simulink model "TestModeleMachineElectrique"  (Simulink 10.0)
settings: Solver=VariableStepAuto  StartTime=0.0  StopTime=10.0  RelTol=1e-3
values from neighbouring files (symbols this model uses):
  ess_coulombic_eff = 0.99    [Batteries.m]
  ess_max_ah_cap = 28    [Batteries.m]
  ess_module_number = 20    [Batteries.m]
  ess_r = [0.01266 0.00685	0.00644	0.00599	0.00587	0.00575	0.00568	0.00581	0.00623	0.00667  0.00635]    [Batteries.m]
  ess_soc = [0:.1:1]    [Batteries.m]
  ess_tau = 0.1    [Batteries.m]
  ess_voc = [12.5 12.8 13.1 13.3 13.4 13.4 13.5 13.6 13.7 13.9 14.2]    [Batteries.m]
  mc_eff_map = 0.01*[ 20	20	20	20	20	20	20	20	20	20	20	20	20	20	20	20	20	20	20	20	20 ... (first row only)    [MachineElectrique.m]
  mc_inertia = 0.0226    [MachineElectrique.m]
  mc_map_spd = [0 500 1000 1500 2000 2500 3000 4000 5000 6000 7000]*(2*pi)/60    [MachineElectrique.m]
  mc_max_trq = [512 508.1 504.2 500.3 496.3	492.4 488.5 480.7 472.8 465 0]    *4.448/3.281/12    [MachineElectrique.m]
  mc_min_trq = -1*[512 508.1 504.2 500.3 496.3	492.4 488.5 480.7 472.8 465 0]    *4.448/3.281/12    [MachineElectrique.m]
  SocInit = 0.8    [Batteries.m]
settings Model: Creator=szhang6_  LastModifiedBy=szhang6_
settings DataIOCC: SaveFormat=Dataset
settings OptimizationCC: LifeSpan=auto
settings DebuggingCC: UnderspecifiedInitializationDetection=Simplified  MergeDetectMultiDrivingBlocksExec=error  SFUnexpectedBacktrackingDiag=error  SFNoUnconditionalDefaultTransitionDiag=error  SFExecutionAtInitializationDiag=warning  ArithmeticOperatorsInVariantConditions=error
settings HardwareCC: ProdBitPerPointer=64  ProdBitPerSizeT=64  ProdBitPerPtrDiffT=64  ProdLargestAtomicFloat=Float  ProdIntDivRoundTo=Zero  ProdEndianess=LittleEndian  ProdWordSize=64  ProdHWDeviceType=Intel->x86-64 (Windows64)
settings ModelReferenceCC: PropagateSignalLabelsOutOfModel=on
settings SFSimCC: SimUseLocalCustomCode=on  CustomCodeUndefinedFunction=FilterOut
settings RTWCC: RTWUseLocalCustomCode=on
settings CodeAppCC: StateflowObjectComments=off
settings GRTTargetCC: TargetLangStandard=C99 (ISO)  CombineOutputUpdateFcns=on  GRTInterface=off
settings ConfigComp: CovMetricSettings=dwe  CovHtmlReporting=off  CovSaveCumulativeToWorkspaceVar=off  CovSaveSingleToWorkspaceVar=off

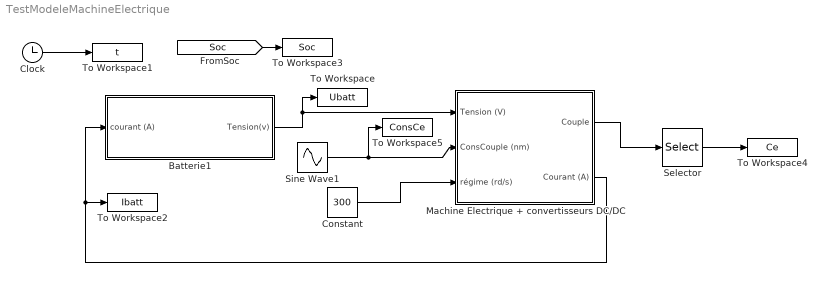
== system TestModeleMachineElectrique ==
  Batterie1 : Subsystem
  Clock : Clock
  Constant : Constant  Value=300
  Machine Electrique + convertisseurs DC/DC : Subsystem
  Selector : Selector  InputPortWidth=2  IndexOptions=Index vector (dialog)  Indices=1  OutputSizes=1
  Sine Wave1 : Sin  Amplitude=100  Frequency=pi  SampleTime=0
  To Workspace : ToWorkspace  VariableName=Ubatt  SampleTime=-1
  To Workspace1 : ToWorkspace  VariableName=t  SampleTime=-1
  To Workspace2 : ToWorkspace  VariableName=Ibatt  SampleTime=-1
  To Workspace3 : ToWorkspace  VariableName=Soc  SampleTime=-1
  To Workspace4 : ToWorkspace  VariableName=Ce  SampleTime=-1
  To Workspace5 : ToWorkspace  VariableName=ConsCe  SampleTime=-1
  wires:
  Machine Electrique + convertisseurs DC/DC/1(Couple) -> Selector/1
  Machine Electrique + convertisseurs DC/DC/2(Courant (A)) -> Batterie1/1(courant (A)), To Workspace2/1
  Constant/1 -> Machine Electrique + convertisseurs DC/DC/3(régime (rd/s))
  Batterie1/1(Tension(v)) -> Machine Electrique + convertisseurs DC/DC/1(Tension (V)), To Workspace/1
  Selector/1 -> To Workspace4/1
  Clock/1 -> To Workspace1/1
  [Soc] -> To Workspace3/1
  Sine Wave1/1 -> Machine Electrique + convertisseurs DC/DC/2(ConsCouple (nm)), To Workspace5/1

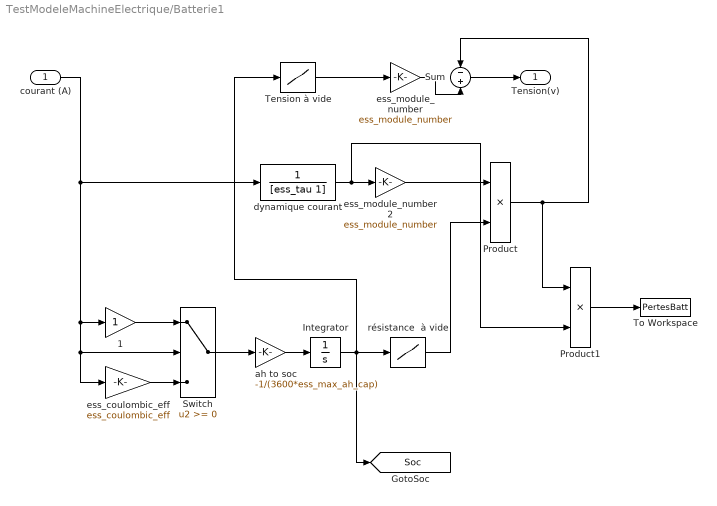
== system TestModeleMachineElectrique/Batterie1 ==
  courant (A) : Inport
  1 : Gain
  Integrator : Integrator  InitialCondition=SocInit
  Product : Product  Inputs=**
  Product1 : Product  Inputs=**
  Sum : Sum  Inputs=-+
  Switch : Switch
  Tension à vide : Lookup  InputValues=ess_soc  Table=ess_voc
  To Workspace : ToWorkspace  VariableName=PertesBatt  SampleTime=-1
  "ah to soc " : Gain  Gain=-1/(3600*ess_max_ah_cap)
  dynamique courant : TransferFcn  Denominator=[ess_tau 1]
  "ess_coulombic_eff " : Gain  Gain=ess_coulombic_eff
  "ess_module_number " : Gain  Gain=ess_module_number
  ess_module_number 2 : Gain  Gain=ess_module_number
  résistance  à vide : Lookup  InputValues=ess_soc  Table=ess_r
  Tension(v) : Outport
  tag scope: Soc=global
  wires:
  courant (A)/1 -> dynamique courant/1, "ess_coulombic_eff "/1, Switch/2, 1/1
  1/1 -> Switch/1
  "ess_coulombic_eff "/1 -> Switch/3
  Switch/1 -> "ah to soc "/1
  "ah to soc "/1 -> Integrator/1
  dynamique courant/1 -> Product1/2, ess_module_number 2/1
  Integrator/1 -> Tension à vide/1, résistance  à vide/1, [Soc]
  ess_module_number 2/1 -> Product/1
  résistance  à vide/1 -> Product/2
  Product/1 -> Product1/1, Sum/1
  Sum/1 -> Tension(v)/1
  Tension à vide/1 -> "ess_module_number "/1
  "ess_module_number "/1 -> Sum/2
  Product1/1 -> To Workspace/1

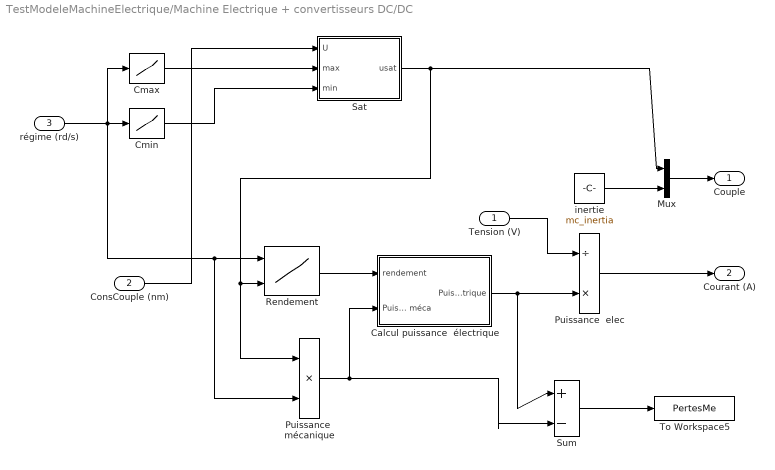
== system TestModeleMachineElectrique/Machine Electrique + convertisseurs DC/DC ==
  Tension (V) : Inport
  ConsCouple (nm) : Inport  Port=2
  régime (rd/s) : Inport  Port=3
  Calcul puissance  électrique : Subsystem
  Cmax : Lookup  InputValues=mc_map_spd  Table=mc_max_trq
  Cmin : Lookup  InputValues=mc_map_spd  Table=mc_min_trq
  Mux : Mux  Inputs=2
  "Puissance  elec " : Product  Inputs=/*
  Puissance  mécanique : Product  Inputs=**
  Rendement : Lookup2D  RowIndex=mc_map_spd  ColumnIndex=mc_map_trq  Table=mc_eff_map  SaturateOnIntegerOverflow=on  InputSameDT=on
  Sat : Subsystem
  Sum : Sum  Inputs=|+-
  To Workspace5 : ToWorkspace  VariableName=PertesMe  SampleTime=-1
  inertie : Constant  Value=mc_inertia
  Couple : Outport
  Courant (A) : Outport  Port=2
  wires:
  régime (rd/s)/1 -> Puissance  mécanique/2, Rendement/1, Cmax/1, Cmin/1
  Rendement/1 -> Calcul puissance  électrique/1(rendement)
  Mux/1 -> Couple/1
  "Puissance  elec "/1 -> Courant (A)/1
  inertie/1 -> Mux/2
  ConsCouple (nm)/1 -> Sat/1(U)
  Cmax/1 -> Sat/2(max)
  Cmin/1 -> Sat/3(min)
  Tension (V)/1 -> "Puissance  elec "/1
  Sat/1(usat) -> Rendement/2, Puissance  mécanique/1, Mux/1
  Sum/1 -> To Workspace5/1
  Calcul puissance  électrique/1(Puissance électrique) -> Sum/1, "Puissance  elec "/2
  Puissance  mécanique/1 -> Sum/2, Calcul puissance  électrique/2(Puissance méca)

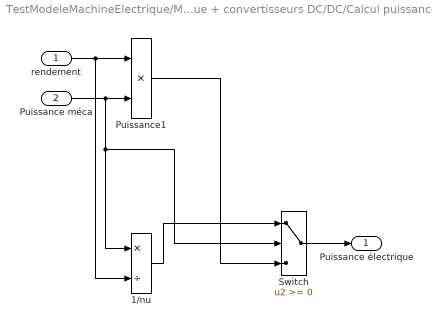
== system TestModeleMachineElectrique/Machine Electrique + convertisseurs DC/DC/Calcul puissance  électrique ==
  rendement : Inport
  Puissance méca : Inport  Port=2
  1/nu : Product  Inputs=*/
  Puissance1 : Product  Inputs=**
  Switch : Switch
  Puissance électrique : Outport
  wires:
  rendement/1 -> 1/nu/2, Puissance1/1
  Puissance1/1 -> Switch/3
  1/nu/1 -> Switch/1
  Switch/1 -> Puissance électrique/1
  Puissance méca/1 -> 1/nu/1, Switch/2, Puissance1/2

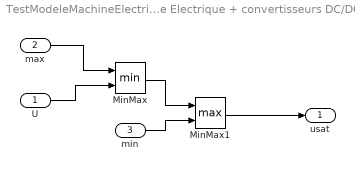
== system TestModeleMachineElectrique/Machine Electrique + convertisseurs DC/DC/Sat ==
  U : Inport
  max : Inport  Port=2
  min : Inport  Port=3
  MinMax : MinMax  Inputs=2
  MinMax1 : MinMax  Function=max  Inputs=2
  usat : Outport
  wires:
  max/1 -> MinMax/1
  U/1 -> MinMax/2
  MinMax/1 -> MinMax1/1
  min/1 -> MinMax1/2
  MinMax1/1 -> usat/1
